simulink model "sim_car_model3"  (R2022a)
settings: Solver=VariableStepAuto  StartTime=0.0  StopTime=70  RelTol=1e-3
values from neighbouring files (symbols this model uses):
  b = (Fmax - c*Vmax^2)/Vmax    (= 2.52478421655)    [Copy_of_script.m]    (also in script.m)
  c = 0.5*rho*A*cd    (= 0.4907934)    [Copy_of_script.m]    (also in script.m)
  Fmax = Pmax/Vmax    (= 1173.27449102)    [Copy_of_script.m]    (also in script.m)
  g = 9.82    [Copy_of_script.m]    (also in script.m)
  m = 1001    [Copy_of_script.m]    (also in script.m)
libraries: slpidlib x1
settings Model: Creator=gomag  LastModifiedBy=gomag

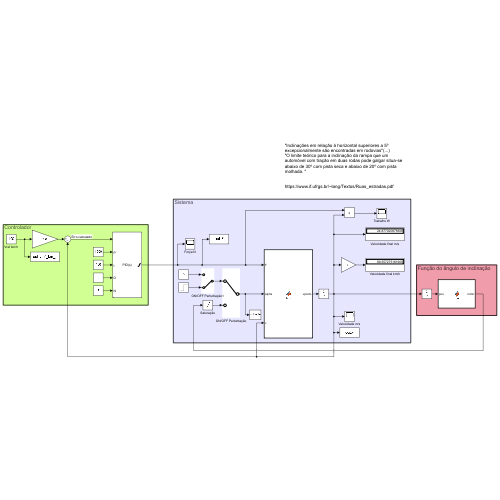
[thumbnail: Simulink's stored preview of the top-level diagram]
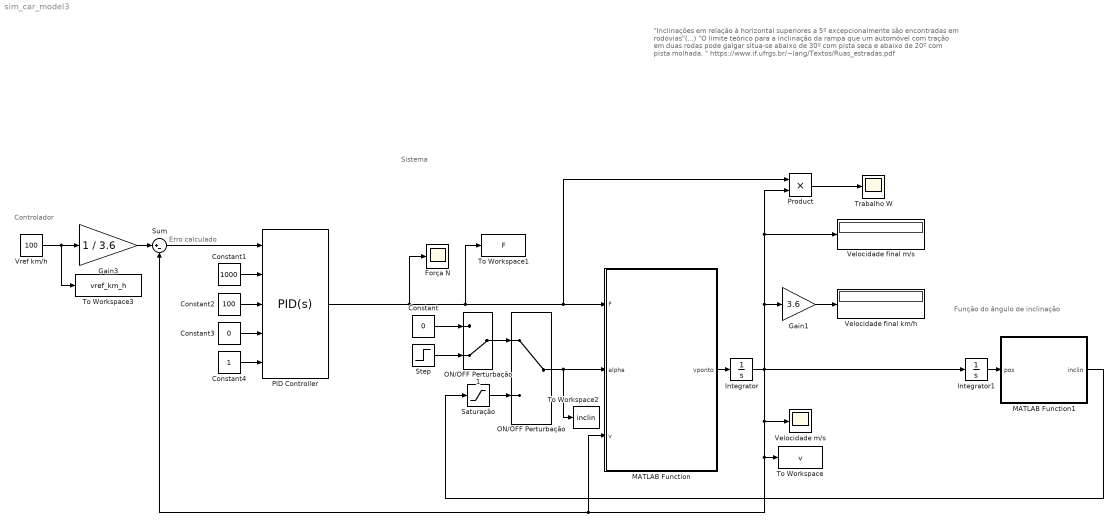
== system sim_car_model3 ==
  note: Controlador
  note: Função do ângulo de inclinação
  note: Sistema
  note: "Inclinações em relação à horizontal superiores a 5º excepcionalmente são encontradas em rodovias"(...)
      | "O limite teórico para a inclinação da rampa que um automóvel com tração em duas rodas pode galgar situa-se abaixo de 30º com pista seca e abaixo de 20º com pista molhada. "
      |
      | https://www.if.ufrgs.br/~lang/Textos/Ruas_estradas.pdf
  note: Erro calculado
  Constant : Constant  Value=0
  Constant1 : Constant  Value=1000
  Constant2 : Constant  Value=100
  Constant3 : Constant  Value=0
  Constant4 : Constant
  Força N : Scope
  Gain1 : Gain  Gain=3.6
  Gain3 : Gain  Gain=1 / 3.6
  Integrator : Integrator
  Integrator1 : Integrator
  MATLAB Function : MATLAB Function  TreatAsAtomicUnit=on
  MATLAB Function1 : MATLAB Function  TreatAsAtomicUnit=on
  ON/OFF Perturbação : ManualSwitch
  ON/OFF Perturbação1 : ManualSwitch  CurrentSetting=0
  PID Controller : slpidlib/PID Controller  Controller=PID  Form=Parallel  TimeDomain=Continuous-time  UseExternalTs=off  SampleTime=-1  IntegratorMethod=Forward Euler  FilterMethod=Forward Euler  ControllerParametersSource=external  P=1000  I=100  UseKiTs=off  D=0  N=100  UseFilter=on  TunerSelectOption=Transfer Function Based (PID Tuner App)  InitialConditionSource=internal  InitialConditionForIntegrator=0  InitialConditionForFilter=0  DifferentiatorICPrevScaledInput=0  ExternalReset=none  TrackingMode=off  Kt=1  LimitOutput=on  SatLimitsSource=internal  UpperSaturationLimit=Fmax  LowerSaturationLimit=-200  LinearizeAsGain=on  AntiWindupMode=clamping  Kb=1  POutMin=[]  POutMax=[]  IOutMin=[]  IOutMax=[]  DOutMin=[]  DOutMax=[]  NOutMin=[]  NOutMax=[]  SumOutMin=[]  SumOutMax=[]  SaturationOutMin=[]  SaturationOutMax=[]  PParamMin=[]  PParamMax=[]  IParamMin=[]  IParamMax=[]  DParamMin=[]  DParamMax=[]  NParamMin=[]  NParamMax=[]  KbParamMin=[]  KbParamMax=[]  KtParamMin=[]  KtParamMax=[]  KbOutMin=[]  KbOutMax=[]  KtOutMin=[]  KtOutMax=[]  IntegratorOutMin=[]  IntegratorOutMax=[]  FilterOutMin=[]  FilterOutMax=[]  SumI1OutMin=[]  SumI1OutMax=[]  SumI2OutMin=[]  SumI2OutMax=[]  SumI3OutMin=[]  SumI3OutMax=[]  SumI4OutMin=[]  SumI4OutMax=[]  SumDOutMin=[]  SumDOutMax=[]  DifferentiatorOutMin=[]  DifferentiatorOutMax=[]  FilterDiffOutCoefMin=[]  FilterDiffOutCoefMax=[]  ReciprocalOutMin=[]  ReciprocalOutMax=[]  SumDenOutMin=[]  SumDenOutMax=[]  SumNumOutMin=[]  SumNumOutMax=[]  DivideOutMin=[]  DivideOutMax=[]  UdiffTsProdOutMin=[]  UdiffTsProdOutMax=[]  NTsProdOutMin=[]  NTsProdOutMax=[]  UintegralTsProdOutMin=[]  UintegralTsProdOutMax=[]  UngainTsProdOutMin=[]  UngainTsProdOutMax=[]  IntegratorContinuousStateAttributes=''  IntegratorStateMustResolveToSignalObject=off  IntegratorRTWStateStorageClass=Auto  FilterContinuousStateAttributes=''  FilterStateMustResolveToSignalObject=off  FilterRTWStateStorageClass=Auto  ParallelPVariant=ExternalParameters  IdealPVariant=Disabled  IVariant=ExternalParameters  DVariant=ExternalParameters  IntegratorVariant=Continuous  SatVariant=Enabled  AWVariant=ContClampingParallel  PCopyVariant=Disabled  TRVariant=Disabled  FdbkBlocksVariant=Forward  IdealPFdbkVariant=Disabled  SatFdbkVariant=Disabled  DerivativeFilterVariant=ContFilter  NVariant=ExternalParameters  NCopyVariant=Disabled  FilterICVariant=InternalICsFilter  IntegratorICVariant=InternalICs  ExternalResetVariant=Disabled  TRSumVariant=Passthrough  SumFdbkVariant=Disabled  SumVariant=Sum_PID  TsampFilterVariant=InternalTs  TsampNgainVariant=Passthrough  TsampIntegralVariant=Passthrough  ExternalSaturationOutDataTypeStr=Inherit: Same as second input  aMode=0
  Product : Product
  Saturação : Saturate  UpperLimit=5*pi/180  LowerLimit=-5*pi/180
  Step : Step  Time=40  After=5*pi/180  SampleTime=0
  Sum : Sum  Inputs=|+-
  To Workspace : ToWorkspace  VariableName=v  SaveFormat=Timeseries  SampleTime=-1
  To Workspace1 : ToWorkspace  VariableName=F  SaveFormat=Timeseries  SampleTime=-1
  To Workspace2 : ToWorkspace  VariableName=inclin  SaveFormat=Timeseries  SampleTime=-1
  To Workspace3 : ToWorkspace  VariableName=vref_km_h  SaveFormat=Timeseries  SampleTime=-1
  Trabalho W : Scope
  Velocidade final km/h : Display
      settings: Decimation=4
  Velocidade final m/s : Display
      settings: Decimation=4
  Velocidade m/s : Scope
  Vref km/h : Constant  Value=100
  wires:
  MATLAB Function/1(vponto) -> Integrator/1
  Product/1 -> Trabalho W/1
  Gain1/1 -> Velocidade final km/h/1
  Integrator1/1 -> MATLAB Function1/1(pos)
  Saturação/1 -> ON/OFF Perturbação/2
  Sum/1 -> PID Controller/1
  Integrator/1 -> Integrator1/1, Gain1/1, Velocidade final m/s/1, Product/2, Velocidade m/s/1, To Workspace/1, MATLAB Function/3(v), Sum/2
  Gain3/1 -> Sum/1
  MATLAB Function1/1(inclin) -> Saturação/1
  Vref km/h/1 -> To Workspace3/1, Gain3/1
  ON/OFF Perturbação/1 -> MATLAB Function/2(alpha), To Workspace2/1
  PID Controller/1 -> MATLAB Function/1(F), Product/1, To Workspace1/1, Força N/1
  ON/OFF Perturbação1/1 -> ON/OFF Perturbação/1
  Step/1 -> ON/OFF Perturbação1/2
  Constant/1 -> ON/OFF Perturbação1/1
  Constant4/1 -> PID Controller/5
  Constant3/1 -> PID Controller/4
  Constant2/1 -> PID Controller/3
  Constant1/1 -> PID Controller/2

== matlab function sim_car_model3/MATLAB Function1 ==
  data: pos input; inclin output; freq_ang_rota parameter
function inclin = fcn(pos,freq_ang_rota)

%Atenuador de frequencia
aten=200;

%Parametros
freq= freq_ang_rota / aten;
amp= 0.1;

%Função
inclin = amp*sin(pos * freq);

== matlab function sim_car_model3/MATLAB Function ==
  data: F input; vponto output; alpha input; v input; b parameter; c parameter; m parameter; g parameter
function vponto = fcn(F, alpha, v, b, c, m, g)

vponto=( F - b*v - c*v^2 - m*g*sin(alpha) ) / m;
